simulink model "Hardware_in_the_Loop_2019a"  (R2021a)
settings: Solver=FixedStepAuto  StartTime=0.0  StopTime=inf  FixedStep=1e-3  RelTol=1e-3  EnableMultiTasking=on
undefined symbols (not defined in the file): k
libraries: arduinolib x3, eeGeneralControl x2
settings Model: FPTRunName=Active  SILPILModeSetting=veronly  ExtModeTrigDuration=2  Creator=ronid  LastModifiedBy=User
settings SolverCC: AlgebraicLoopSolver=TrustRegion  AutoInsertRateTranBlk=on
settings DataIOCC: LimitDataPoints=on  SaveFormat=Array
settings OptimizationCC: ExpressionDepthLimit=2147483647  LifeSpan=Inf  MaxStackSize=64
settings DebuggingCC: UnderspecifiedInitializationDetection=Classic  MergeDetectMultiDrivingBlocksExec=none  ParameterPrecisionLossMsg=none  FcnCallInpInsideContextMsg=warning  AllowSymbolicDim=off  StateNameClashWarn=warning  SFUnexpectedBacktrackingDiag=warning  SFNoUnconditionalDefaultTransitionDiag=warning  SFExecutionAtInitializationDiag=none  SFMachineParentedDataDiag=warning  ArithmeticOperatorsInVariantConditions=warning
settings HardwareCC: ProdBitPerInt=16  ProdBitPerPointer=16  ProdBitPerSizeT=16  ProdBitPerPtrDiffT=16  ProdLargestAtomicFloat=None  ProdWordSize=8  ProdHWDeviceType=Atmel->AVR  UseEmbeddedCoderFeatures=off
settings ModelReferenceCC: PropagateSignalLabelsOutOfModel=off
settings SFSimCC: SimUseLocalCustomCode=off  CustomCodeUndefinedFunction=UseInterfaceOnly
settings RTWCC: SystemTargetFile=ert.tlc  HardwareBoard=Arduino Mega 2560  TemplateMakefile=ert_default_tmf  GenerateReport=on  RTWVerbose=off  RTWUseLocalCustomCode=off  Toolchain=Arduino AVR  BuildConfiguration=Faster Runs  LaunchReport=on
settings CodeAppCC: ForceParamTrailComments=on  OperatorAnnotations=on  StateflowObjectComments=on  MATLABSourceComments=on
settings ERTTargetCC: MultiwordLength=2048  ERTCustomFileBanners=off  SupportContinuousTime=on  SupportNonInlinedSFcns=on  RemoveResetFunc=off  SupportVariableSizeSignals=on  ModelStepFunctionPrototypeControlCompliant=off  ExtModeStaticAllocSize=2048
settings ConfigComp: CovMetricSettings=dw  CovSaveCumulativeToWorkspaceVar=on  CovSaveSingleToWorkspaceVar=on  CovExternalEMLEnable=off  CovSFcnEnable=off

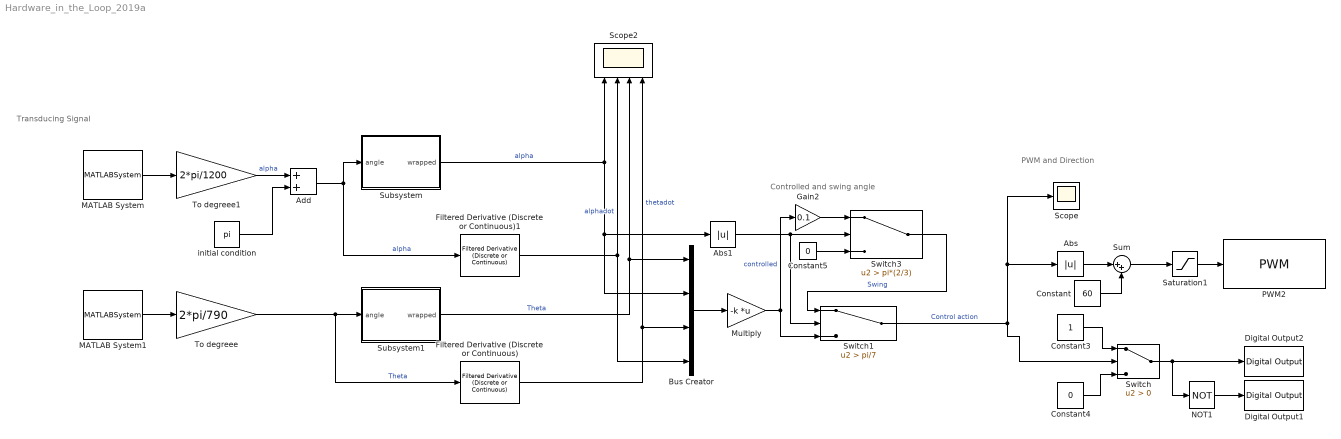
== system Hardware_in_the_Loop_2019a ==
  note: Controlled and swing angle
  note: Transducing Signal
  note: PWM and Direction
  Abs : Abs  OutDataTypeStr=double
  Abs1 : Abs  OutDataTypeStr=double
  Add : Sum  AccumDataTypeStr=double
  Bus Creator : BusCreator  Inputs=4
  Constant : Constant  Value=60
  Constant3 : Constant
  Constant4 : Constant  Value=0
  Constant5 : Constant  Value=0
  Digital Output1 : arduinolib/Digital Output  pinNumber=8  Direction=output  blockPlatform=arduino
  Digital Output2 : arduinolib/Digital Output  pinNumber=7  Direction=output  blockPlatform=arduino
  Filtered Derivative (Discrete or Continuous) : eeGeneralControl/Filtered Derivative (Discrete or Continuous)  K=1  T=0.001  B=inf  A=-inf  minRatio=10  init_option=Inherited from block input  x0=0  Ts=0.001
      settings: SourceProductBaseCode=PS
  Filtered Derivative (Discrete or Continuous)1 : eeGeneralControl/Filtered Derivative (Discrete or Continuous)  K=1  T=0.001  B=inf  A=-inf  minRatio=10  init_option=Inherited from block input  x0=0  Ts=0.001
      settings: SourceProductBaseCode=PS
  Gain2 : Gain  Gain=0.1  OutDataTypeStr=double
  MATLAB System : MATLABSystem  System=Encoder_arduino_3  Encoder=1  PinA=3  PinB=5  SampleTime=0.001
      mask Type: Encoder_arduino_3
      mask Display:
      | disp('Encoder');
      | port_label('output',1,'y');
  MATLAB System1 : MATLABSystem  System=Encoder_arduino_2  Encoder=0  PinA=2  PinB=4  SampleTime=0.001
      mask Type: Encoder_arduino_2
      mask Display:
      | disp('Encoder');
      | port_label('output',1,'y');
  Multiply : Gain  Gain=-k  Multiplication=Matrix(K*u) (u vector)  OutDataTypeStr=double
  NOT1 : Logic  Operator=NOT  IconShape=distinctive  AllPortsSameDT=off  OutDataTypeStr=boolean
  PWM2 : arduinolib/PWM  pinNumber=6  frequencyType=Default  desiredFrequency=490.2  achievableFrequency=490.2
  Saturation1 : Saturate  UpperLimit=255  LowerLimit=0
  Scope : Scope
  Scope2 : Scope  NumInputPorts=4
  Subsystem : Subsystem
  Subsystem1 : Subsystem
  Sum : Sum  Inputs=|++
  Switch : Switch  Criteria=u2 > Threshold  OutDataTypeStr=double
  Switch1 : Switch  Criteria=u2 > Threshold  Threshold=pi/7  OutDataTypeStr=double
  Switch3 : Switch  Criteria=u2 > Threshold  Threshold=pi*(2/3)  OutDataTypeStr=double
  To degreee : Gain  Gain=2*pi/790  OutDataTypeStr=double
  To degreee1 : Gain  Gain=2*pi/1200  OutDataTypeStr=double
  initial condition : Constant  Value=pi
  wires:
  Filtered Derivative (Discrete or Continuous)/1 -> Bus Creator/3, Scope2/4  "thetadot"
  MATLAB System1/1 -> To degreee/1
  Filtered Derivative (Discrete or Continuous)1/1 -> Bus Creator/4, Scope2/2  "alphadot"
  Subsystem/1(wrapped) -> Abs1/1, Bus Creator/2, Scope2/1  "alpha"
  MATLAB System/1 -> To degreee1/1
  Switch/1 -> NOT1/1, Digital Output2/1
  Constant4/1 -> Switch/3
  NOT1/1 -> Digital Output1/1
  Constant3/1 -> Switch/1
  Saturation1/1 -> PWM2/1
  Bus Creator/1 -> Multiply/1
  Subsystem1/1(wrapped) -> Bus Creator/1, Scope2/3  "Theta"
  Add/1 -> Filtered Derivative (Discrete or Continuous)1/1, Subsystem/1(angle)  "alpha"
  Abs1/1 -> Switch1/2, Switch3/2
  To degreee/1 -> Filtered Derivative (Discrete or Continuous)/1, Subsystem1/1(angle)  "Theta"
  initial condition/1 -> Add/2
  To degreee1/1 -> Add/1  "alpha"
  Gain2/1 -> Switch3/1
  Switch3/1 -> Switch1/1  "Swing"
  Multiply/1 -> Switch1/3, Gain2/1  "controlled"
  Constant5/1 -> Switch3/3
  Abs/1 -> Sum/1
  Sum/1 -> Saturation1/1
  Constant/1 -> Sum/2
  Switch1/1 -> Switch/2, Abs/1, Scope/1  "Control action"

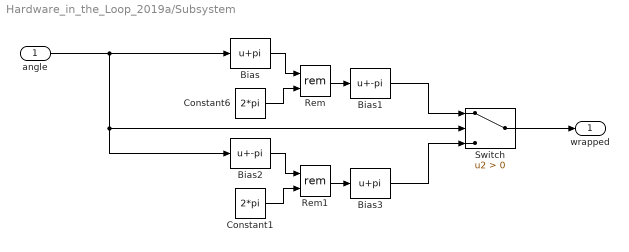
== system Hardware_in_the_Loop_2019a/Subsystem ==
  angle : Inport
  Bias : Bias  Bias=pi
  Bias1 : Bias  Bias=-pi
  Bias2 : Bias  Bias=-pi
  Bias3 : Bias  Bias=pi
  Constant1 : Constant  Value=2*pi
  Constant6 : Constant  Value=2*pi
  Rem : Math  Operator=rem  SignedPower=on  SaturateOnIntegerOverflow=on
  Rem1 : Math  Operator=rem  SignedPower=on  SaturateOnIntegerOverflow=on
  Switch : Switch  Criteria=u2 > Threshold  OutDataTypeStr=double
  wrapped : Outport
  wires:
  Constant6/1 -> Rem/2
  Bias1/1 -> Switch/1
  Bias/1 -> Rem/1
  Rem/1 -> Bias1/1
  Bias3/1 -> Switch/3
  Rem1/1 -> Bias3/1
  angle/1 -> Switch/2, Bias2/1, Bias/1
  Constant1/1 -> Rem1/2
  Bias2/1 -> Rem1/1
  Switch/1 -> wrapped/1

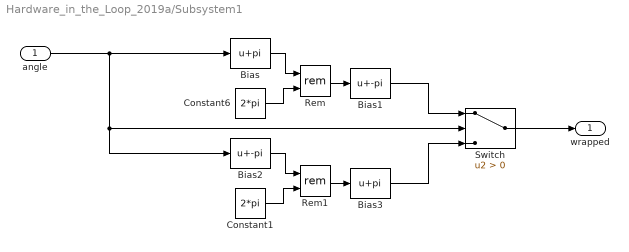
== system Hardware_in_the_Loop_2019a/Subsystem1 ==
  angle : Inport
  Bias : Bias  Bias=pi
  Bias1 : Bias  Bias=-pi
  Bias2 : Bias  Bias=-pi
  Bias3 : Bias  Bias=pi
  Constant1 : Constant  Value=2*pi
  Constant6 : Constant  Value=2*pi
  Rem : Math  Operator=rem  SignedPower=on  SaturateOnIntegerOverflow=on
  Rem1 : Math  Operator=rem  SignedPower=on  SaturateOnIntegerOverflow=on
  Switch : Switch  Criteria=u2 > Threshold  OutDataTypeStr=double
  wrapped : Outport
  wires:
  Constant6/1 -> Rem/2
  Bias1/1 -> Switch/1
  Bias/1 -> Rem/1
  Rem/1 -> Bias1/1
  Bias3/1 -> Switch/3
  Rem1/1 -> Bias3/1
  angle/1 -> Switch/2, Bias2/1, Bias/1
  Constant1/1 -> Rem1/2
  Bias2/1 -> Rem1/1
  Switch/1 -> wrapped/1
